simulink model "SWP_LQR_tracking"  (R2021a)
settings: Solver=ode4  StartTime=0.0  StopTime=500  FixedStep=1e-3  RelTol=1e-3
settings Model: Creator=aarti  LastModifiedBy=aarti

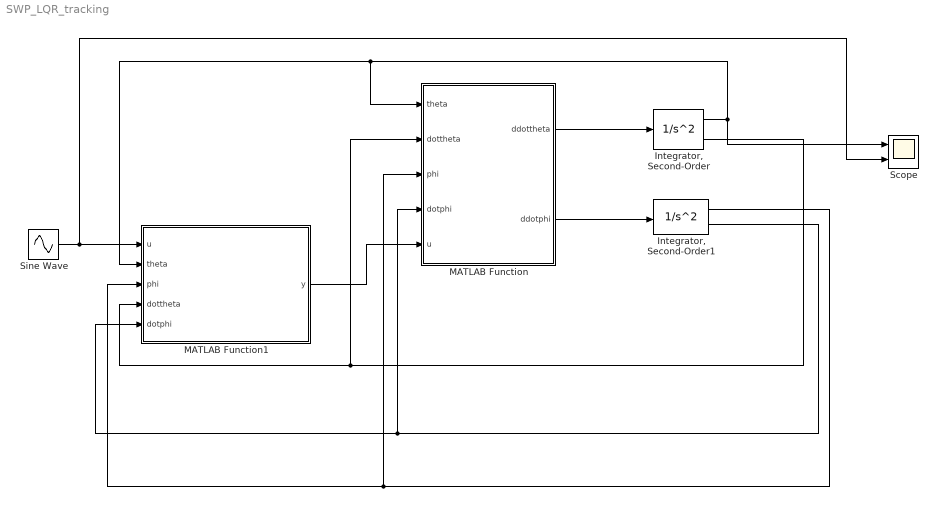
== system SWP_LQR_tracking ==
  "Integrator, Second-Order" : SecondOrderIntegrator  WrapX=on
  "Integrator, Second-Order1" : SecondOrderIntegrator  WrapX=on
  MATLAB Function : MATLAB Function  TreatAsAtomicUnit=on
  MATLAB Function1 : MATLAB Function  TreatAsAtomicUnit=on
  Scope : Scope  NumInputPorts=2
  Sine Wave : Sin  Amplitude=0.1  Frequency=0.01  SampleTime=0
  wires:
  MATLAB Function/1(ddottheta) -> "Integrator, Second-Order"/1
  "Integrator, Second-Order"/1 -> MATLAB Function/1(theta), MATLAB Function1/2(theta), Scope/1
  "Integrator, Second-Order"/2 -> MATLAB Function/2(dottheta), MATLAB Function1/4(dottheta)
  MATLAB Function/2(ddotphi) -> "Integrator, Second-Order1"/1
  "Integrator, Second-Order1"/2 -> MATLAB Function/4(dotphi), MATLAB Function1/5(dotphi)
  MATLAB Function1/1(y) -> MATLAB Function/5(u)
  "Integrator, Second-Order1"/1 -> MATLAB Function/3(phi), MATLAB Function1/3(phi)
  Sine Wave/1 -> Scope/2, MATLAB Function1/1(u)

== matlab function SWP_LQR_tracking/MATLAB Function1 ==
  data: u input; y output; theta input; phi input; dottheta input; dotphi input
function y = fcn(u, theta, phi, dottheta, dotphi)
    K = [-8.5622    2.4574    0.3115    0.6764] ;
    y = -K*[theta - u; phi ; dottheta ; dotphi] - 1  ;
end

== matlab function SWP_LQR_tracking/MATLAB Function ==
  data: theta input; dottheta input; phi input; dotphi input; u input; ddottheta output; ddotphi output
function [ddottheta,ddotphi]=SwirlingPendulum(theta,dottheta,phi,dotphi,u)
%% Swirling Pendulum Equations of Motion
% Define the parameter values
m1 = 0.6976; m2 = 0.086; l1 = 0.0519; l2 =0.065; g = 9.81;
g = 9.81;
% Inertia Matrix
M=[4/3*(m1*l1^2+m2*(3*l1^2+(l2*sin(phi))^2)), 2*m2*l1*l2*cos(phi);
    2*m2*l1*l2*cos(phi), 4/3*(m2*l2^2)];
% Coriolis 
C=[0 8/3*(m2*l2^2)*sin(phi)*cos(phi)*dottheta-2*m2*l1*l2*sin(phi)*dotphi;-4/3*m2*l2^2*cos(phi)*sin(phi)*dottheta 0];
% Potential Terms
G=[(m1+2*m2)*g*l1*sin(theta)+m2*g*l2*sin(phi)*cos(theta);
    m2*g*l2*sin(theta)*cos(phi)];
B=[0;1];
%Mx''+Cx'+G=Bu;
ddotX=inv(M)*(-C*[dottheta;dotphi]-G+B*u);
ddottheta=ddotX(1,:);
ddotphi=ddotX(2,:);
